simulink model "Factorial_ForLoop"  (R2021a)
settings: Solver=FixedStepDiscrete  StartTime=0.0  StopTime=1  RelTol=1e-3
settings Model: Creator=Moamen_Hamed  LastModifiedBy=Mahmoud Shams El-Din
settings OptimizationCC: DefaultParameterBehavior=Inlined  EnhancedBackFolding=on  PassReuseOutputArgsAs=Individual arguments  OptimizeBlockOrder=speed  DifferentSizesBufferReuse=on  OptimizationCustomize=off  EfficientTunableParamExpr=on
settings DebuggingCC: ParameterTunabilityLossMsg=error
settings SFSimCC: MATLABDynamicMemAlloc=off
settings RTWCC: SystemTargetFile=ert.tlc  GenCodeOnly=on  TemplateMakefile=ert_default_tmf  GenerateReport=on  IncludeHyperlinkInReport=on  LaunchReport=on  GenerateTraceInfo=on
settings CodeAppCC: ForceParamTrailComments=on  IgnoreCustomStorageClasses=off  OperatorAnnotations=on  SimulinkDataObjDesc=on  SFDataObjDesc=on  InsertBlockDesc=on
settings ERTTargetCC: TargetLangStandard=C99 (ISO)  GenerateSampleERTMain=on  CodeInterfacePackaging=Reusable function  SupportComplex=off  InlinedParameterPlacement=NonHierarchical  ERTCustomFileTemplate=example_file_process.tlc

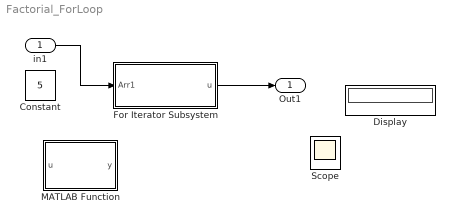
== system Factorial_ForLoop ==
  in1 : Inport  PortDimensions=1
  Constant : Constant  Value=5  OutDataTypeStr=uint32
  Display : Display
  For Iterator Subsystem : Subsystem  TreatAsAtomicUnit=on
  MATLAB Function : MATLAB Function  TreatAsAtomicUnit=on
  Scope : Scope  NumInputPorts=2
  Out1 : Outport
  wires:
  in1/1 -> For Iterator Subsystem/1(Arr1)
  For Iterator Subsystem/1(u) -> Out1/1

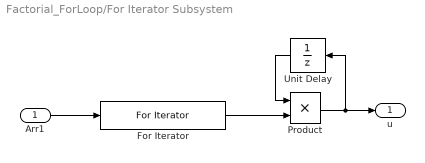
== system Factorial_ForLoop/For Iterator Subsystem ==
  Arr1 : Inport
  For Iterator : ForIterator  IterationSource=external  IterationVariableDataType=uint32
  Product : Product  OutDataTypeStr=uint32
  Unit Delay : UnitDelay  InitialCondition=1  SampleTime=-1  HasFrameUpgradeWarning=on
  u : Outport
  wires:
  For Iterator/1 -> Product/2
  Arr1/1 -> For Iterator/1
  Unit Delay/1 -> Product/1
  Product/1 -> Unit Delay/1, u/1

== matlab function Factorial_ForLoop/MATLAB Function ==
  data: u input; y output
function y = Factorial(u)

y = factorial(u);
